simulink library "pmm"  (R2021b)
settings: Solver=VariableStepAuto  StartTime=0.0  StopTime=10.0  RelTol=1e-3
undefined symbols (not defined in the file or in its folder): ENUM_ACMAINRLYSTS_OPEN, ENUM_ACPRECHRGRLYSTS_OPEN, ENUM_B2VRLYSTA_OPEN, ENUM_BMSHVSTS_HVOPEN, ENUM_BRAKEPEDAL_RELEASED, ENUM_CACRLYDEM_CLOSE, ENUM_CACRLYSTS_OPEN, ENUM_CHRGFAULT_ACRLYFAIL, ENUM_CHRGFAULT_BCUHVFAIL, ENUM_CHRGFAULT_BCUNEGFAIL, ENUM_CHRGFAULT_BCUTIMEOUT, ENUM_CHRGFAULT_DCDCENABLE, ENUM_CHRGFAULT_DCDCRLYFAIL, ENUM_CHRGFAULT_HVILFAIL, ENUM_CHRGFAULT_PDUHVFAIL, ENUM_CHRGFAULT_RLYCHKFAIL, ENUM_DCDCEACPCURLYSTA_CLOSED, ENUM_DCDCEACPCURLYSTA_FAILTOCLOSE, ENUM_DCDCEACPCURLYSTA_OPEN, ENUM_DCDCEACPCURLYSTA_WELDED, ENUM_DCDCENABLESTS_READY, ENUM_DCDCRLYSTS_OPEN, ENUM_EHPSRLYDEM_CLOSE, ENUM_EHPSRLYSTS_OPEN, ENUM_FOGRLYENCMD_DISABLE, ENUM_GEARACTUALPOSN_D, ENUM_HVPWROFFREQ_POWEROFF, ENUM_KEYSTATUS_OFF, ENUM_KEYSTATUS_ON, ENUM_KEYSTATUS_START, ENUM_LOWBATTVOLTAGE_NORMAL, ENUM_LOWBATTVOLTAGE_POWERDOWN, ENUM_LOWBATTVOLTAGE_POWERUP, ENUM_MCUHVLOOP_POWEROFF, ENUM_MCUHVLOOPSTS_OPEN, ENUM_MCUMAINRLYSTS_OPEN, ENUM_MCUPRECHRGRLYSTS_OPEN, ENUM_PDFAULT_ACRLYOPEN, ENUM_PDFAULT_BCUDISABLE, ENUM_PDFAULT_DCDCDISABLE, ENUM_PDFAULT_DCDCRLYOPEN, ENUM_PDFAULT_EACDISABLE, ENUM_PDFAULT_EACRLYOPEN, ENUM_PDFAULT_EHPSDISABLE, ENUM_PDFAULT_EHPSRLYOPEN, ENUM_PDFAULT_MCUDISABLE, ENUM_PDFAULT_MCUDISCHRG, ENUM_PDFAULT_MCURLYOPEN, ENUM_PEUSELFCHKSTS_NOFAULT, ENUM_PLUGINSTS_NOPLUGIN, ENUM_PLUGINSTS_PLUGIN, ENUM_PMMMODE_DRIVE, ENUM_PMMMODE_LVBATCHRG, ENUM_PUSTATE_DCDCENABLE, ENUM_PUSTATE_EACPRESCHECK, ENUM_PUSTATE_EHPSENABLE, ENUM_PUSTATE_MCUENABLE, ENUM_PUSTATE_PDUMCURLYCLOSED, ENUM_PUSTATE_POWERUPFAIL, ENUM_TARGETGEAR_REVERSE ... (+126)
libraries: hcu_lib x45, simulink x5, ddm x1, dsc x1
(part 3 of 7)

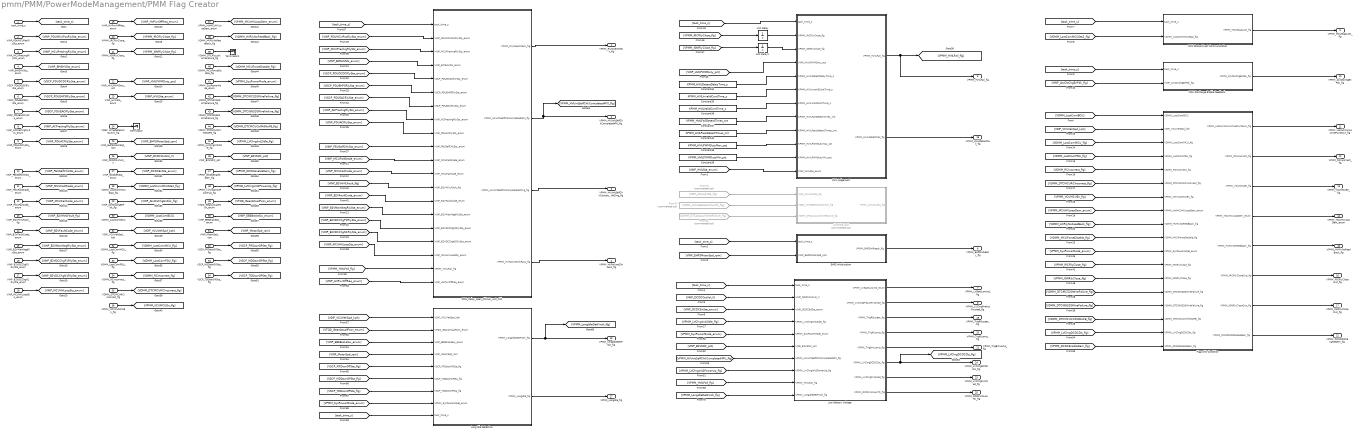
== system pmm/PMM/PowerModeManagement/PMM Flag Creator  ==
  task_time_s : Inport
  VINP_PDUMCUPosRlySta_enum : Inport  Port=2
  VINP_MCUPrechrgRlySts_enum : Inport  Port=3
  VINP_BMSHVSts_enum : Inport  Port=4
  VSCP_PDUDCDCRlySta_enum : Inport  Port=5
  VSCP_PDUEHPSRlySta_enum : Inport  Port=6
  VSCP_PDUEACRlySta_enum : Inport  Port=7
  VINP_ACPrechrgRlySts_enum : Inport  Port=8
  VINP_PDUACRlySta_enum : Inport  Port=9
  VINP_PEUSelfChkSts_enum : Inport  Port=10
  VINP_MCUFailGrade_enum : Inport  Port=11
  VINP_MCUFailCode_enum : Inport  Port=12
  VINP_B2VHVILFault_flg : Inport  Port=13
  VINP_B2VFaultCode_enum : Inport  Port=14
  VINP_B2VMainNegRlySta_enum : Inport  Port=15
  VINP_B2VDCChgP1RlySta_enum : Inport  Port=16
  VINP_B2VDCChgN1RlySta_enum : Inport  Port=17
  VINP_MCUHVLoopSts_enum : Inport  Port=18
  VINP_HVPwrOffReq_enum : Inport  Port=19
  VPMM_IRCRlyClose_flg : Inport  Port=20
  VPMM_IGNRlyClose_flg : Inport  Port=21
  VINP_HVILPWMDuty_pct : Inport  Port=22
  VINP_HVILSta_enum : Inport  Port=23
  VDSC_WineDetectorSwitch_flg : Inport  Port=24
  VINP_EHPSMotorSpd_rpm : Inport  Port=25
  VINP_DCDCOutVol_V : Inport  Port=26
  VINP_DCDCEnSta_enum : Inport  Port=27
  VDMM_LostComMCUSta2_flg : Inport  Port=28
  VINP_AtvDisChgEnFbk_flg : Inport  Port=29
  VDMM_LostComBCU : Inport  Port=30
  VDIP_VCUVehSpd_kph : Inport  Port=31
  VDMM_LostComMCU_flg : Inport  Port=32
  VDMM_LostComPDU_flg : Inport  Port=33
  VDMM_RCIncorrect_flg : Inport  Port=34
  VDMM_DTCMCURCIncorrect_flg : Inport  Port=35
  VPMM_InitVCUMCUEn_flg : Inport  Port=36
  VPMM_InitMCUHVLoopDem_enum : Inport  Port=37
  VDMM_HVRlyNoFeedBack_flg : Inport  Port=38
  VDMM_DTCAlcLockWireFailure_flg : Inport  Port=39
  VDMM_MCUForceDisable_flg : Inport  Port=40
  VPMM_SysPowerMode_enum : Inport  Port=41
  VDMM_DTCIRCS2GWireFailure_flg : Inport  Port=42
  VDMM_DTCIGNS2GWireFailure_flg : Inport  Port=43
  VDMM_DTCMCUCtrlMdNoFB_flg : Inport  Port=44
  VPMM_LVChrgIinit2Idle_flg : Inport  Port=45
  VINP_B2VSOC_pct : Inport  Port=46
  VPMM_DCDCEnableDem_flg : Inport  Port=47
  VPMM_LVChrgInit2PowerUp_flg : Inport  Port=48
  VTQD_GearActualPosn_enum : Inport  Port=49
  VINP_EBSBrakeSw_enum : Inport  Port=50
  VINP_MotorSpd_rpm : Inport  Port=51
  VSCP_FRDoorOPSta_flg : Inport  Port=52
  VSCP_MDDoorOPSta_flg : Inport  Port=53
  VSCP_TDDoorOPSta_flg : Inport  Port=54
  "Alcohole Lock " : Subsystem  Commented=on
  Constant34 : Constant  Value=KPMM_HVILDetectDelayTime_s
  Constant35 : Constant  Value=KPMM_HVILInvalidContTime_s
  Constant36 : Constant  Value=KPMM_HVILValidContTime_s
  Constant37 : Constant  Value=KPMM_HVILFailDetectTimes_cnt
  Constant38 : Constant  Value=KPMM_HVILPWMDutyMax_pct
  Constant39 : Constant  Value=KPMM_HVILPWMDutyMin_pct
  Constant40 : Constant  Value=KPMM_HVILPassDetectTimes_cnt
  EHPS Initialization : Subsystem
  Flag with Condition : Subsystem
  From24 : From  Commented=on  GotoTag=VDMM_DTCAlcLockWireFailure_flg
  From73 : From  Commented=on  GotoTag=VINP_AlcLockSta_flg
  From74 : From  Commented=on  GotoTag=VDSC_WineDetectorSwitch_flg
  HVIL Judgement : Subsystem
  Long Idle Detection : Subsystem
  Low Battery Voltage : Subsystem
  MCU Discharge Enable Feedback : Subsystem
  MCU Status2 Lost Communication : Subsystem
  PMM_Relay_open_Chk/HV_unit_Chk : Subsystem  Priority=1
      settings: AttributesFormatString=< Priority = %<Priority>>
  Terminator : Terminator
  Terminator1 : Terminator
  Unit Delay : UnitDelay  SampleTime=-1  HasFrameUpgradeWarning=on
  Unit Delay1 : UnitDelay  SampleTime=-1  HasFrameUpgradeWarning=on
  VPMM_RlyOpenCheck_flg : Outport
  VPMM_HVUnitSelfChkCompleted4PU_flg : Outport  Port=2
  VPMM_HVUnitSelfChkCompleted4Chrg_flg : Outport  Port=3
  VPMM_HVFailureChkPass_flg : Outport  Port=4
  VPMM_HVILFail_flg : Outport  Port=5  VectorParamsAs1DForOutWhenUnconnected=off
  VPMM_EHPSIniReady_flg : Outport  Port=6  VectorParamsAs1DForOutWhenUnconnected=off
  VPMM_LVBattLowInd_flg : Outport  Port=7
  VPMM_LVChrgPreActFinished_flg : Outport  Port=8
  VPMM_MCUSta2Lost_flg : Outport  Port=9  VectorParamsAs1DForOutWhenUnconnected=off
  VPMM_AtvDisChgEnFbk_flg : Outport  Port=10  VectorParamsAs1DForOutWhenUnconnected=off
  VPMM_LostHVComActivePwrDown_flg : Outport  Port=11
  VPMM_RCIncorrect_flg : Outport  Port=12  VectorParamsAs1DForOutWhenUnconnected=off
  VPMM_VCUMCUEn_flg : Outport  Port=13  VectorParamsAs1DForOutWhenUnconnected=off
  VPMM_MCUHVLoopDem_enum : Outport  Port=14  VectorParamsAs1DForOutWhenUnconnected=off
  VPMM_HVRlyNoFeedBack_flg : Outport  Port=15  VectorParamsAs1DForOutWhenUnconnected=off
  VPMM_IRCRlyCloseOut_flg : Outport  Port=16  VectorParamsAs1DForOutWhenUnconnected=off
  VPMM_IGNRlyCloseOut_flg : Outport  Port=17  VectorParamsAs1DForOutWhenUnconnected=off
  VPMM_HVILDetectFail_flg : Outport  Port=18  VectorParamsAs1DForOutWhenUnconnected=off
  VPMM_TrigRBuzeer_flg : Outport  Port=19
  VPMM_TrigRLamp_flg : Outport  Port=20
  VPMM_TrigBrkLamp_flg : Outport  Port=21
  VPMM_PMMDCDCEnableDem_flg : Outport  Port=22  VectorParamsAs1DForOutWhenUnconnected=off
  VPMM_LVChrgFinished_flg : Outport  Port=23
  VPMM_LVChrgDCDCDis_flg : Outport  Port=24
  VPMM_DCDCVolLowTO_flg : Outport  Port=25
  VPMM_LongIdleDetFinsh_flg : Outport  Port=26
  VPMM_LongIdle_flg : Outport  Port=27
  wires:
  HVIL Judgement/2(VPMM_HVILDetectFail_flg) -> VPMM_HVILDetectFail_flg/1
  [VINP_B2VHVILFault_flg] -> PMM_Relay_open_Chk/HV_unit_Chk/13(VINP_B2VHVILFault_flg)
  [task_time_s] -> PMM_Relay_open_Chk/HV_unit_Chk/1(task_time_s)
  [VINP_PEUSelfChkSts_enum] -> PMM_Relay_open_Chk/HV_unit_Chk/10(VINP_PEUSelfChkSts_enum)
  [VPMM_HVILFail_flg] -> PMM_Relay_open_Chk/HV_unit_Chk/19(VPMM_HVILFail_flg)
  [VINP_MCUHVLoopSts_enum] -> PMM_Relay_open_Chk/HV_unit_Chk/18(VINP_MCUHVLoopSts_enum)
  [VINP_B2VMainNegRlySta_enum] -> PMM_Relay_open_Chk/HV_unit_Chk/15(VINP_B2VMainNegRlySta_enum)
  [VINP_B2VFaultCode_enum] -> PMM_Relay_open_Chk/HV_unit_Chk/14(VINP_B2VFaultCode_enum)
  [VINP_B2VDCChgN1RlySta_enum] -> PMM_Relay_open_Chk/HV_unit_Chk/17(VINP_B2VDCChgN1RlySta_enum)
  [VINP_HVPwrOffReq_enum] -> PMM_Relay_open_Chk/HV_unit_Chk/20(VINP_HVPwrOffReq_enum)
  [VINP_B2VDCChgP1RlySta_enum] -> PMM_Relay_open_Chk/HV_unit_Chk/16(VINP_B2VDCChgP1RlySta_enum)
  [VINP_PDUACRlySta_enum] -> PMM_Relay_open_Chk/HV_unit_Chk/9(VINP_PDUACRlySta_enum)
  [VINP_MCUPrechrgRlySts_enum] -> PMM_Relay_open_Chk/HV_unit_Chk/3(VINP_MCUPrechrgRlySts_enum)
  PMM_Relay_open_Chk/HV_unit_Chk/3(VPMM_HVUnitSelfChkCompleted4Chrg_flg) -> VPMM_HVUnitSelfChkCompleted4Chrg_flg/1
  [VSCP_PDUEACRlySta_enum] -> PMM_Relay_open_Chk/HV_unit_Chk/7(VSCP_PDUEACRlySta_enum)
  [VINP_BMSHVSts_enum] -> PMM_Relay_open_Chk/HV_unit_Chk/4(VINP_BMSHVSts_enum)
  [VSCP_PDUDCDCRlySta_enum] -> PMM_Relay_open_Chk/HV_unit_Chk/5(VSCP_PDUDCDCRlySta_enum)
  [VINP_PDUMCUPosRlySta_enum] -> PMM_Relay_open_Chk/HV_unit_Chk/2(VINP_PDUMCUPosRlySta_enum)
  [VINP_ACPrechrgRlySts_enum] -> PMM_Relay_open_Chk/HV_unit_Chk/8(VINP_ACPrechrgRlySts_enum)
  [VSCP_PDUEHPSRlySta_enum] -> PMM_Relay_open_Chk/HV_unit_Chk/6(VSCP_PDUEHPSRlySta_enum)
  [VINP_MCUFailGrade_enum] -> PMM_Relay_open_Chk/HV_unit_Chk/11(VINP_MCUFailGrade_enum)
  PMM_Relay_open_Chk/HV_unit_Chk/1(VPMM_RlyOpenCheck_flg) -> VPMM_RlyOpenCheck_flg/1
  PMM_Relay_open_Chk/HV_unit_Chk/2(VPMM_HVUnitSelfChkCompleted4PU_flg) -> [VPMM_HVUnitSelfChkCompleted4PU_flg], VPMM_HVUnitSelfChkCompleted4PU_flg/1
  [VINP_MCUFailCode_enum] -> PMM_Relay_open_Chk/HV_unit_Chk/12(VINP_MCUFailCode_enum)
  PMM_Relay_open_Chk/HV_unit_Chk/4(VPMM_HVFailureChkPass_flg) -> VPMM_HVFailureChkPass_flg/1
  task_time_s/1 -> [task_time_s]
  VINP_PDUMCUPosRlySta_enum/1 -> [VINP_PDUMCUPosRlySta_enum]
  VINP_MCUPrechrgRlySts_enum/1 -> [VINP_MCUPrechrgRlySts_enum]
  VINP_BMSHVSts_enum/1 -> [VINP_BMSHVSts_enum]
  VSCP_PDUDCDCRlySta_enum/1 -> [VSCP_PDUDCDCRlySta_enum]
  VSCP_PDUEHPSRlySta_enum/1 -> [VSCP_PDUEHPSRlySta_enum]
  VSCP_PDUEACRlySta_enum/1 -> [VSCP_PDUEACRlySta_enum]
  VINP_ACPrechrgRlySts_enum/1 -> [VINP_ACPrechrgRlySts_enum]
  VINP_PDUACRlySta_enum/1 -> [VINP_PDUACRlySta_enum]
  VINP_PEUSelfChkSts_enum/1 -> [VINP_PEUSelfChkSts_enum]
  VINP_MCUFailGrade_enum/1 -> [VINP_MCUFailGrade_enum]
  VINP_MCUFailCode_enum/1 -> [VINP_MCUFailCode_enum]
  VINP_B2VHVILFault_flg/1 -> [VINP_B2VHVILFault_flg]
  VINP_B2VFaultCode_enum/1 -> [VINP_B2VFaultCode_enum]
  VINP_B2VMainNegRlySta_enum/1 -> [VINP_B2VMainNegRlySta_enum]
  VINP_B2VDCChgP1RlySta_enum/1 -> [VINP_B2VDCChgP1RlySta_enum]
  VINP_B2VDCChgN1RlySta_enum/1 -> [VINP_B2VDCChgN1RlySta_enum]
  VINP_MCUHVLoopSts_enum/1 -> [VINP_MCUHVLoopSts_enum]
  VINP_HVPwrOffReq_enum/1 -> [VINP_HVPwrOffReq_enum]
  [task_time_s] -> HVIL Judgement/1(task_time_s)
  [VPMM_IRCRlyClose_flg] -> Unit Delay/1
  Unit Delay1/1 -> HVIL Judgement/3(VPMM_IGNRlyClose_flg)
  [VPMM_IGNRlyClose_flg] -> Unit Delay1/1
  [VINP_HVILPWMDuty_pct] -> HVIL Judgement/4(VINP_HVILPWMDuty_pct)
  Constant36/1 -> HVIL Judgement/7(KPMM_HVILValidContTime_s)
  Constant40/1 -> HVIL Judgement/9(KPMM_HVILPassDetectTimes_cnt)
  Constant37/1 -> HVIL Judgement/8(KPMM_HVILFailDetectTimes_cnt)
  Unit Delay/1 -> HVIL Judgement/2(VPMM_IRCRlyClose_flg)
  Constant35/1 -> HVIL Judgement/6(KPMM_HVILInvalidContTime_s)
  Constant38/1 -> HVIL Judgement/10(KPMM_HVILPWMDutyMax_pct)
  Constant34/1 -> HVIL Judgement/5(KPMM_HVILDetectDelayTime_s)
  Constant39/1 -> HVIL Judgement/11(KPMM_HVILPWMDutyMin_pct)
  HVIL Judgement/1(VPMM_HVILFail_flg) -> [VPMM_HVILFail_flg], VPMM_HVILFail_flg/1
  [VINP_HVILSta_enum] -> HVIL Judgement/12(VINP_HVILSta_enum)
  VPMM_IRCRlyClose_flg/1 -> [VPMM_IRCRlyClose_flg]
  VPMM_IGNRlyClose_flg/1 -> [VPMM_IGNRlyClose_flg]
  VINP_HVILPWMDuty_pct/1 -> [VINP_HVILPWMDuty_pct]
  VINP_HVILSta_enum/1 -> [VINP_HVILSta_enum]
  From73/1 -> "Alcohole Lock "/1(VINP_AlcLockSta_flg)
  From74/1 -> "Alcohole Lock "/2(VDSC_WineDetectorSwitch_flg)
  VDSC_WineDetectorSwitch_flg/1 -> Terminator/1
  EHPS Initialization/1(VPMM_EHPSIniReady_flg) -> VPMM_EHPSIniReady_flg/1
  [task_time_s] -> EHPS Initialization/1(task_time_s)
  [VINP_EHPSMotorSpd_rpm] -> EHPS Initialization/2(VINP_EHPSMotorSpd_rpm)
  VINP_EHPSMotorSpd_rpm/1 -> [VINP_EHPSMotorSpd_rpm]
  Low Battery Voltage/1(VPMM_LVBattLowInd_enum) -> VPMM_LVBattLowInd_flg/1
  [task_time_s] -> Low Battery Voltage/1(task_time_s)
  VINP_DCDCEnSta_enum/1 -> [VINP_DCDCEnSta_enum]
  VINP_DCDCOutVol_V/1 -> [VINP_DCDCOutVol_V]
  [VINP_DCDCOutVol_V] -> Low Battery Voltage/2(VINP_DCDCOutVol_V)
  [VINP_DCDCEnSta_enum] -> Low Battery Voltage/3(VINP_DCDCEnSta_enum)
  MCU Status2 Lost Communication/1(VPMM_MCUSta2Lost_flg) -> VPMM_MCUSta2Lost_flg/1
  VDMM_LostComMCUSta2_flg/1 -> [VDMM_LostComMCUSta2_flg]
  [task_time_s] -> MCU Status2 Lost Communication/1(task_time_s)
  [VDMM_LostComMCUSta2_flg] -> MCU Status2 Lost Communication/2(VDMM_LostComMCUSta2_flg)
  MCU Discharge Enable Feedback/1(VPMM_AtvDisChgEnFbk_flg) -> VPMM_AtvDisChgEnFbk_flg/1
  [task_time_s] -> MCU Discharge Enable Feedback/1(task_time_s)
  [VINP_AtvDisChgEnFbk_flg] -> MCU Discharge Enable Feedback/2(VINP_AtvDisChgEnFbk_flg)
  VINP_AtvDisChgEnFbk_flg/1 -> [VINP_AtvDisChgEnFbk_flg]
  Flag with Condition/1(VPMM_LostHVComActivePwrDown_flg) -> VPMM_LostHVComActivePwrDown_flg/1
  Flag with Condition/2(VPMM_RCIncorrect_flg) -> VPMM_RCIncorrect_flg/1
  Flag with Condition/3(VPMM_VCUMCUEn_flg) -> VPMM_VCUMCUEn_flg/1
  Flag with Condition/4(VPMM_MCUHVLoopDem_enum) -> VPMM_MCUHVLoopDem_enum/1
  VDMM_LostComBCU/1 -> [VDMM_LostComBCU]
  VDMM_DTCMCURCIncorrect_flg/1 -> [VDMM_DTCMCURCIncorrect_flg]
  VDMM_LostComPDU_flg/1 -> [VDMM_LostComPDU_flg]
  VPMM_InitVCUMCUEn_flg/1 -> [VPMM_VCUMCUEn_flg]
  VPMM_InitMCUHVLoopDem_enum/1 -> [VPMM_MCUHVLoopDem_enum]
  VDMM_LostComMCU_flg/1 -> [VDMM_LostComMCU_flg]
  VDMM_RCIncorrect_flg/1 -> [VDMM_RCIncorrect_flg]
  VDIP_VCUVehSpd_kph/1 -> [VDIP_VCUVehSpd_kph]
  [VDMM_LostComBCU] -> Flag with Condition/1(VDMM_LostComBCU)
  [VDIP_VCUVehSpd_kph] -> Flag with Condition/2(VDIP_VCUVehSpd_kph)
  [VDMM_LostComMCU_flg] -> Flag with Condition/3(VDMM_LostComMCU_flg)
  [VDMM_LostComPDU_flg] -> Flag with Condition/4(VDMM_LostComPDU_flg)
  [VDMM_RCIncorrect_flg] -> Flag with Condition/5(VDMM_RCIncorrect_flg)
  [VDMM_DTCMCURCIncorrect_flg] -> Flag with Condition/6(VDMM_DTCMCURCIncorrect_flg)
  [VPMM_VCUMCUEn_flg] -> Flag with Condition/7(VPMM_InitVCUMCUEn_flg)
  [VPMM_MCUHVLoopDem_enum] -> Flag with Condition/8(VPMM_InitMCUHVLoopDem_enum)
  [VDMM_HVRlyNoFeedBack_flg] -> Flag with Condition/9(VDMM_HVRlyNoFeedBack_flg)
  Flag with Condition/5(VPMM_HVRlyNoFeedBack_flg) -> VPMM_HVRlyNoFeedBack_flg/1
  VDMM_HVRlyNoFeedBack_flg/1 -> [VDMM_HVRlyNoFeedBack_flg]
  From24/1 -> "Alcohole Lock "/3(VDMM_DTCAlcLockWireFailure_flg)
  VDMM_DTCAlcLockWireFailure_flg/1 -> Terminator1/1
  VDMM_MCUForceDisable_flg/1 -> [VDMM_MCUForceDisable_flg]
  [VDMM_MCUForceDisable_flg] -> Flag with Condition/10(VDMM_MCUForceDisable_flg)
  VPMM_SysPowerMode_enum/1 -> [VPMM_SysPowerMode_enum]
  [VPMM_SysPowerMode_enum] -> Flag with Condition/11(VPMM_SysPowerMode_enum)
  VDMM_DTCIRCS2GWireFailure_flg/1 -> [VDMM_DTCIRCS2GWireFailure_flg]
  VDMM_DTCIGNS2GWireFailure_flg/1 -> [VDMM_DTCIGNS2GWireFailure_flg]
  Flag with Condition/6(VPMM_IRCRlyCloseOut_flg) -> VPMM_IRCRlyCloseOut_flg/1
  Flag with Condition/7(VPMM_IGNRlyCloseOut_flg) -> VPMM_IGNRlyCloseOut_flg/1
  [VPMM_IRCRlyClose_flg] -> Flag with Condition/12(VPMM_IRCRlyClose_flg)
  [VPMM_IGNRlyClose_flg] -> Flag with Condition/13(VPMM_IGNRlyClose_flg)
  [VDMM_DTCIRCS2GWireFailure_flg] -> Flag with Condition/14(VDMM_DTCIRCS2GWireFailure_flg)
  [VDMM_DTCIGNS2GWireFailure_flg] -> Flag with Condition/15(VDMM_DTCIGNS2GWireFailure_flg)
  VDMM_DTCMCUCtrlMdNoFB_flg/1 -> [VDMM_DTCMCUCtrlMdNoFB_flg]
  [VDMM_DTCMCUCtrlMdNoFB_flg] -> Flag with Condition/16(VDMM_DTCMCUCtrlMdNoFB_flg)
  Low Battery Voltage/2(VPMM_LVChrgPreActFinished_flg) -> VPMM_LVChrgPreActFinished_flg/1
  [VPMM_LVChrgIinit2Idle_flg] -> Low Battery Voltage/4(VPMM_LVChrgIinit2Idle_flg)
  VPMM_LVChrgIinit2Idle_flg/1 -> [VPMM_LVChrgIinit2Idle_flg]
  [VPMM_SysPowerMode_enum] -> Low Battery Voltage/5(VPMM_SysPowerMode_enum)
  Low Battery Voltage/5(VPMM_TrigBrkLamp_flg) -> VPMM_TrigBrkLamp_flg/1
  Low Battery Voltage/4(VPMM_TrigRLamp_flg) -> VPMM_TrigRLamp_flg/1
  Low Battery Voltage/3(VPMM_TrigRBuzeer_flg) -> VPMM_TrigRBuzeer_flg/1
  [VINP_B2VSOC_pct] -> Low Battery Voltage/6(VINP_B2VSOC_pct)
  VINP_B2VSOC_pct/1 -> [VINP_B2VSOC_pct]
  [VPMM_HVUnitSelfChkCompleted4PU_flg] -> Low Battery Voltage/7(VPMM_HVUnitSelfChkCompleted4PU_flg)
  Low Battery Voltage/6(VPMM_LVChrgDCDCDis_flg) -> [VPMM_LVChrgDCDCDis_flg], VPMM_LVChrgDCDCDis_flg/1
  [VPMM_LVChrgDCDCDis_flg] -> Flag with Condition/17(VPMM_LVChrgDCDCDis_flg)
  VPMM_DCDCEnableDem_flg/1 -> [VPMM_DCDCEnableDem_flg]
  [VPMM_DCDCEnableDem_flg] -> Flag with Condition/18(VPMM_DCDCEnableDem_flg)
  Flag with Condition/8(VPMM_PMMDCDCEnableDem_flg) -> VPMM_PMMDCDCEnableDem_flg/1
  Low Battery Voltage/7(VPMM_LVChrgFinished_flg) -> VPMM_LVChrgFinished_flg/1
  Low Battery Voltage/8(VPMM_DCDCVolLowTO_flg) -> VPMM_DCDCVolLowTO_flg/1
  VPMM_LVChrgInit2PowerUp_flg/1 -> [VPMM_LVChrgInit2PowerUp_flg]
  [VPMM_LVChrgInit2PowerUp_flg] -> Low Battery Voltage/8(VPMM_LVChrgInit2PowerUp_flg)
  [VPMM_HVILFail_flg] -> Low Battery Voltage/9(VPMM_HVILFail_flg)
  [VDIP_VCUVehSpd_kph] -> Long Idle Detection/1(VDIP_VCUVehSpd_kph)
  [VTQD_GearActualPosn_enum] -> Long Idle Detection/2(VTQD_GearActualPosn_enum)
  [VINP_EBSBrakeSw_enum] -> Long Idle Detection/3(VINP_EBSBrakeSw_enum)
  [VINP_MotorSpd_rpm] -> Long Idle Detection/4(VINP_MotorSpd_rpm)
  [VSCP_FRDoorOPSta_flg] -> Long Idle Detection/5(VSCP_FRDoorOPSta_flg)
  [VSCP_MDDoorOPSta_flg] -> Long Idle Detection/6(VSCP_MDDoorOPSta_flg)
  [VSCP_TDDoorOPSta_flg] -> Long Idle Detection/7(VSCP_TDDoorOPSta_flg)
  [task_time_s] -> Long Idle Detection/9(task_time_s)
  Long Idle Detection/1(VPMM_LongIdleDetFinsh_flg) -> [VPMM_LongIdleDetFinsh_flg], VPMM_LongIdleDetFinsh_flg/1
  VTQD_GearActualPosn_enum/1 -> [VTQD_GearActualPosn_enum]
  VINP_EBSBrakeSw_enum/1 -> [VINP_EBSBrakeSw_enum]
  VINP_MotorSpd_rpm/1 -> [VINP_MotorSpd_rpm]
  VSCP_FRDoorOPSta_flg/1 -> [VSCP_FRDoorOPSta_flg]
  VSCP_MDDoorOPSta_flg/1 -> [VSCP_MDDoorOPSta_flg]
  VSCP_TDDoorOPSta_flg/1 -> [VSCP_TDDoorOPSta_flg]
  [VPMM_LongIdleDetFinsh_flg] -> Low Battery Voltage/10(VPMM_LongIdleDetFinsh_flg)
  Long Idle Detection/2(VPMM_LongIdle_flg) -> VPMM_LongIdle_flg/1
  [VPMM_SysPowerMode_enum] -> Long Idle Detection/8(VPMM_SysPowerMode_enum)

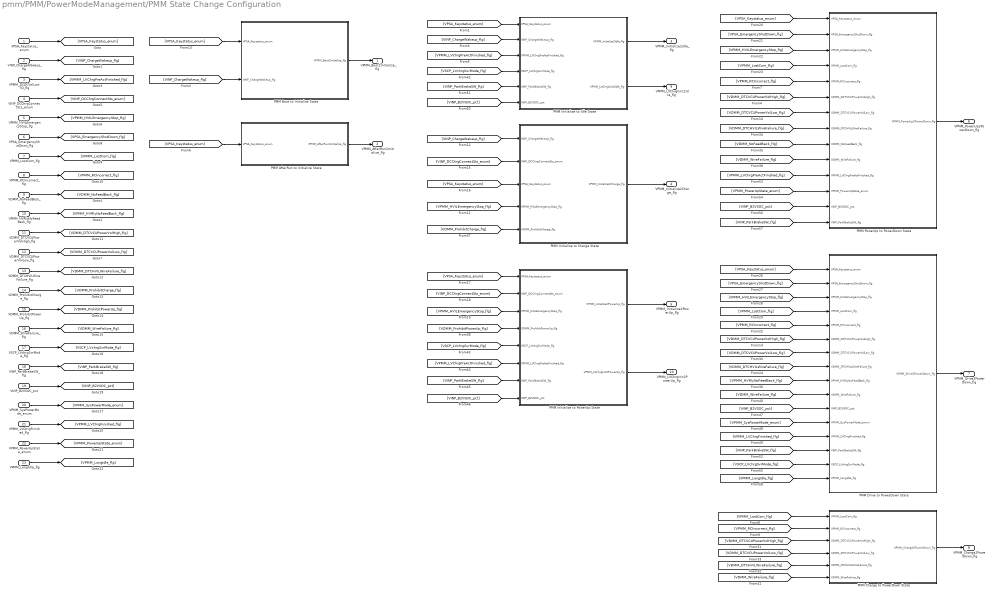
== system pmm/PMM/PowerModeManagement/PMM State Change Configuration ==
  VPSA_Keystatus_enum : Inport
  VINP_ChargeWakeup_flg : Inport  Port=2
  VPMM_DCDCVolLowTO_flg : Inport  Port=3
  VINP_DCChrgConnectSts_enum : Inport  Port=4
  VPMM_HVILEmergencyStop_flg : Inport  Port=5
  VPSA_EmergencyShutDown_flg : Inport  Port=6
  VPMM_LostCom_flg : Inport  Port=7
  VPMM_RCIncorrect_flg : Inport  Port=8
  VDMM_NoFeedBack_flg : Inport  Port=9
  VPMM_HVRlyNoFeedBack_flg : Inport  Port=10
  VDMM_DTCVCUPowerVolHigh_flg : Inport  Port=11
  VDMM_DTCVCUPowerVolLow_flg : Inport  Port=12
  VDMM_DTCHVILWireFailure_flg : Inport  Port=13
  VDMM_ProhibitCharge_flg : Inport  Port=14
  VDMM_ProhibitPowerUp_flg : Inport  Port=15
  VDMM_WireFailure_flg : Inport  Port=16
  VSCP_LVchrgSvrMode_flg : Inport  Port=17
  VINP_ParkBrakeSW_flg : Inport  Port=18
  VINP_B2VSOC_pct : Inport  Port=19
  VPMM_SysPowerMode_enum : Inport  Port=20
  VPMM_LVChrgFinished_flg : Inport  Port=21
  VPMM_PowerUpState_enum : Inport  Port=22
  VPMM_LongIdle_flg : Inport  Port=23
  PMM AfterRun to Initialize State : Subsystem
  PMM Boot to Initialize State : Subsystem
  PMM Charge to PowerDown State : Subsystem
  PMM Drive to PowerDown State : Subsystem
  PMM Initialize to Charge State : Subsystem
  PMM Initialize to Idle State : Subsystem
  PMM Initialize to PowerUp State : Subsystem
  PMM PowerUp to PowerDown State : Subsystem
  VPMM_Boot2Initialize_flg : Outport
  VPMM_AfterRun2Initialize_flg : Outport  Port=2
  VPMM_Initialize2Idle_flg : Outport  Port=3
  VPMM_Initialize2Charge_flg : Outport  Port=4
  VPMM_Initialize2PowerUp_flg : Outport  Port=5
  VPMM_PowerUp2PowerDown_flg : Outport  Port=6
  VPMM_Drive2PowerDown_flg : Outport  Port=7
  VPMM_Charge2PowerDown_flg : Outport  Port=8
  VPMM_LVChrgIinit2Idle_flg : Outport  Port=9
  VPMM_LVChrgInit2PowerUp_flg : Outport  Port=10
  wires:
  [VPSA_EmergencyShutDown_flg] -> PMM PowerUp to PowerDown State/2(VPSA_EmergencyShutDown_flg)
  PMM AfterRun to Initialize State/1(VPMM_AfterRun2Initialize_flg) -> VPMM_AfterRun2Initialize_flg/1
  [VPMM_HVILEmergencyStop_flg] -> PMM Initialize to Charge State/4(VPMM_HVILEmergencyStop_flg)
  PMM Initialize to PowerUp State/1(VPMM_Initialize2PowerUp_flg) -> VPMM_Initialize2PowerUp_flg/1
  [VPSA_EmergencyShutDown_flg] -> PMM Drive to PowerDown State/2(VPSA_EmergencyShutDown_flg)
  [VINP_DCChrgConnectSts_enum] -> PMM Initialize to Charge State/2(VINP_DCChrgConnectSts_enum)
  [VPMM_HVILEmergencyStop_flg] -> PMM PowerUp to PowerDown State/3(VPMM_HVILEmergencyStop_flg)
  [VPMM_LostCom_flg] -> PMM Drive to PowerDown State/4(VPMM_LostCom_flg)
  [VPMM_LostCom_flg] -> PMM Charge to PowerDown State/1(VPMM_LostCom_flg)
  [VINP_ChargeWakeup_flg] -> PMM Initialize to Idle State/2(VINP_ChargeWakeup_flg)
  [VPSA_Keystatus_enum] -> PMM Drive to PowerDown State/1(VPSA_Keystatus_enum)
  PMM Charge to PowerDown State/1(VPMM_Charge2PowerDown_flg) -> VPMM_Charge2PowerDown_flg/1
  [VPMM_HVILEmergencyStop_flg] -> PMM Drive to PowerDown State/3(VPMM_HVILEmergencyStop_flg)
  PMM Boot to Initialize State/1(VPMM_Boot2Initialize_flg) -> VPMM_Boot2Initialize_flg/1
  [VPMM_RCIncorrect_flg] -> PMM Charge to PowerDown State/2(VPMM_RCIncorrect_flg)
  [VPMM_RCIncorrect_flg] -> PMM Drive to PowerDown State/5(VPMM_RCIncorrect_flg)
  [VINP_ChargeWakeup_flg] -> PMM Boot to Initialize State/2(VINP_ChargeWakeup_flg)
  [VPMM_LVChrgPreActFinished_flg] -> PMM Initialize to Idle State/3(VPMM_LVChrgPreActFinished_flg)
  PMM Initialize to Idle State/1(VPMM_Initialize2Idle_flg) -> VPMM_Initialize2Idle_flg/1
  [VPMM_LostCom_flg] -> PMM PowerUp to PowerDown State/4(VPMM_LostCom_flg)
  [VINP_ChargeWakeup_flg] -> PMM Initialize to Charge State/1(VINP_ChargeWakeup_flg)
  [VPSA_Keystatus_enum] -> PMM Initialize to Charge State/3(VPSA_Keystatus_enum)
  PMM Initialize to Charge State/1(VPMM_Initialize2Charge_flg) -> VPMM_Initialize2Charge_flg/1
  [VPMM_HVILEmergencyStop_flg] -> PMM Initialize to PowerUp State/3(VPMM_HVILEmergencyStop_flg)
  [VPSA_Keystatus_enum] -> PMM Boot to Initialize State/1(VPSA_Keystatus_enum)
  PMM Drive to PowerDown State/1(VPMM_Drive2PowerDown_flg) -> VPMM_Drive2PowerDown_flg/1
  [VPSA_Keystatus_enum] -> PMM Initialize to Idle State/1(VPSA_Keystatus_enum)
  [VINP_DCChrgConnectSts_enum] -> PMM Initialize to PowerUp State/2(VINP_DCChrgConnectSts_enum)
  [VPSA_Keystatus_enum] -> PMM Initialize to PowerUp State/1(VPSA_Keystatus_enum)
  [VPSA_Keystatus_enum] -> PMM AfterRun to Initialize State/1(VPSA_Keystatus_enum)
  PMM PowerUp to PowerDown State/1(VPMM_PowerUp2PowerDown_flg) -> VPMM_PowerUp2PowerDown_flg/1
  [VPSA_Keystatus_enum] -> PMM PowerUp to PowerDown State/1(VPSA_Keystatus_enum)
  VPSA_Keystatus_enum/1 -> [VPSA_Keystatus_enum]
  VINP_ChargeWakeup_flg/1 -> [VINP_ChargeWakeup_flg]
  VPMM_DCDCVolLowTO_flg/1 -> [VPMM_LVChrgPreActFinished_flg]
  VINP_DCChrgConnectSts_enum/1 -> [VINP_DCChrgConnectSts_enum]
  VPMM_HVILEmergencyStop_flg/1 -> [VPMM_HVILEmergencyStop_flg]
  VPSA_EmergencyShutDown_flg/1 -> [VPSA_EmergencyShutDown_flg]
  VPMM_LostCom_flg/1 -> [VPMM_LostCom_flg]
  VPMM_RCIncorrect_flg/1 -> [VPMM_RCIncorrect_flg]
  [VPMM_RCIncorrect_flg] -> PMM PowerUp to PowerDown State/5(VPMM_RCIncorrect_flg)
  VPMM_HVRlyNoFeedBack_flg/1 -> [VPMM_HVRlyNoFeedBack_flg]
  VDMM_NoFeedBack_flg/1 -> [VDMM_NoFeedBack_flg]
  VDMM_DTCVCUPowerVolHigh_flg/1 -> [VDMM_DTCVCUPowerVolHigh_flg]
  VDMM_DTCVCUPowerVolLow_flg/1 -> [VDMM_DTCVCUPowerVolLow_flg]
  [VDMM_DTCVCUPowerVolLow_flg] -> PMM PowerUp to PowerDown State/7(VDMM_DTCVCUPowerVolLow_flg)
  [VDMM_DTCVCUPowerVolHigh_flg] -> PMM PowerUp to PowerDown State/6(VDMM_DCTVCUPowerVolHigh_flg)
  VDMM_DTCHVILWireFailure_flg/1 -> [VDMM_DTCHVILWireFailure_flg]
  [VDMM_DTCVCUPowerVolHigh_flg] -> PMM Drive to PowerDown State/6(VDMM_DTCVCUPowerVolHigh_flg)
  [VDMM_DTCVCUPowerVolLow_flg] -> PMM Drive to PowerDown State/7(VDMM_DTCVCUPowerVolLow_flg)
  [VDMM_DTCHVILWireFailure_flg] -> PMM Drive to PowerDown State/8(VDMM_DTCHVILWireFailure_flg)
  [VDMM_DTCVCUPowerVolHigh_flg] -> PMM Charge to PowerDown State/3(VDMM_DTCVCUPowerVolHigh_flg)
  [VDMM_DTCVCUPowerVolLow_flg] -> PMM Charge to PowerDown State/4(VDMM_DTCVCUPowerVolLow_flg)
  [VDMM_DTCHVILWireFailure_flg] -> PMM Charge to PowerDown State/5(VDMM_DTCHVILWireFailure_flg)
  [VDMM_DTCHVILWireFailure_flg] -> PMM PowerUp to PowerDown State/8(VDMM_DTCHVILWireFailure_flg)
  [VDMM_NoFeedBack_flg] -> PMM PowerUp to PowerDown State/9(VDMM_NoFeedBack_flg)
  [VPMM_HVRlyNoFeedBack_flg] -> PMM Drive to PowerDown State/9(VPMM_HVRlyNoFeedBack_flg)
  VDMM_ProhibitCharge_flg/1 -> [VDMM_ProhibitCharge_flg]
  [VDMM_ProhibitCharge_flg] -> PMM Initialize to Charge State/5(VDMM_ProhibitCharge_flg)
  VDMM_ProhibitPowerUp_flg/1 -> [VDMM_ProhibitPowerUp_flg]
  [VDMM_ProhibitPowerUp_flg] -> PMM Initialize to PowerUp State/4(VDMM_ProhibitPowerUp_flg)
  VDMM_WireFailure_flg/1 -> [VDMM_WireFailure_flg]
  [VDMM_WireFailure_flg] -> PMM PowerUp to PowerDown State/10(VDMM_WireFailure_flg)
  [VDMM_WireFailure_flg] -> PMM Drive to PowerDown State/10(VDMM_WireFailure_flg)
  [VDMM_WireFailure_flg] -> PMM Charge to PowerDown State/6(VDMM_WireFailure_flg)
  VSCP_LVchrgSvrMode_flg/1 -> [VSCP_LVchrgSvrMode_flg]
  [VSCP_LVchrgSvrMode_flg] -> PMM Initialize to Idle State/4(VSCP_LVchrgSvrMode_flg)
  PMM Initialize to Idle State/2(VPMM_LVChrgIinit2Idle_flg) -> VPMM_LVChrgIinit2Idle_flg/1
  [VSCP_LVchrgSvrMode_flg] -> PMM Initialize to PowerUp State/5(VSCP_LVchrgSvrMode_flg)
  [VPMM_LVChrgPreActFinished_flg] -> PMM Initialize to PowerUp State/6(VPMM_LVChrgPreActFinished_flg)
  [VINP_B2VSOC_pct] -> PMM Initialize to PowerUp State/8(VINP_B2VSOC_pct)
  [VINP_ParkBrakeSW_flg] -> PMM Initialize to PowerUp State/7(VINP_ParkBrakeSW_flg)
  VINP_ParkBrakeSW_flg/1 -> [VINP_ParkBrakeSW_flg]
  VINP_B2VSOC_pct/1 -> [VINP_B2VSOC_pct]
  PMM Initialize to PowerUp State/2(VPMM_LVChrgInit2PowerUp_flg) -> VPMM_LVChrgInit2PowerUp_flg/1
  [VINP_B2VSOC_pct] -> PMM Drive to PowerDown State/11(VINP_B2VSOC_pct)
  VPMM_SysPowerMode_enum/1 -> [VPMM_SysPowerMode_enum]
  [VPMM_SysPowerMode_enum] -> PMM Drive to PowerDown State/12(VPMM_SysPowerMode_enum)
  VPMM_LVChrgFinished_flg/1 -> [VPMM_LVChrgFinished_flg]
  [VPMM_LVChrgFinished_flg] -> PMM Drive to PowerDown State/13(VPMM_LVChrgFinished_flg)
  [VINP_ParkBrakeSW_flg] -> PMM Initialize to Idle State/5(VINP_ParkBrakeSW_flg)
  [VINP_B2VSOC_pct] -> PMM Initialize to Idle State/6(VINP_B2VSOC_pct)
  [VINP_ParkBrakeSW_flg] -> PMM Drive to PowerDown State/14(VINP_ParkBrakeSW_flg)
  [VPMM_LVChrgPreActFinished_flg] -> PMM PowerUp to PowerDown State/11(VPMM_LVChrgPreActFinished_flg)
  VPMM_PowerUpState_enum/1 -> [VPMM_PowerUpState_enum]
  [VPMM_PowerUpState_enum] -> PMM PowerUp to PowerDown State/12(VPMM_PowerUpState_enum)
  [VSCP_LVchrgSvrMode_flg] -> PMM Drive to PowerDown State/15(VSCP_LVchrgSvrMode_flg)
  [VINP_B2VSOC_pct] -> PMM PowerUp to PowerDown State/13(VINP_B2VSOC_pct)
  [VINP_ParkBrakeSW_flg] -> PMM PowerUp to PowerDown State/14(VINP_ParkBrakeSW_flg)
  VPMM_LongIdle_flg/1 -> [VPMM_LongIdle_flg]
  [VPMM_LongIdle_flg] -> PMM Drive to PowerDown State/16(VPMM_LongIdle_flg)

== system pmm/PMM/PowerModeManagement/PMM Switch Enum Creator ==
  VPMM_InitPowerUpState_enum : Inport
  task_time_s : Inport  Port=2
  VPMM_MCUPrechrgProc_flg : Inport  Port=3
  VPMM_MCUEnableProc_flg : Inport  Port=4
  VPMM_DCDCEnableProc_flg : Inport  Port=5
  VPMM_EHPSEnableProc_flg : Inport  Port=6
  VPMM_CACPresReadyProc_flg : Inport  Port=7
  VPMM_InitPowerDownFault_enum : Inport  Port=8
  VPMM_InitChrgFault_enum : Inport  Port=9
  ChrgFault_SW : Subsystem
  Constant44 : Constant  Value=KPMM_TwoSysSwOFF_flg
  Constant49 : Constant  Value=ENUM_PUSTATE_PDUMCURLYCLOSED
  Constant50 : Constant  Value=ENUM_PUSTATE_MCUENABLE
  Constant51 : Constant  Value=ENUM_PUSTATE_DCDCENABLE
  Constant52 : Constant  Value=ENUM_PUSTATE_EHPSENABLE
  Constant53 : Constant  Value=ENUM_PUSTATE_EACPRESCHECK
  Constant54 : Constant  Value=KPMM_StaSwTime_s
  Data Type Conversion : DataTypeConversion  OutDataTypeStr=uint32
  Data Type Conversion28 : DataTypeConversion
  Data Type Conversion29 : DataTypeConversion
  Data Type Conversion30 : DataTypeConversion
  Divide : Product  Inputs=*/
  Floor : Rounding
  PowerDownFault_SW : Subsystem
  PowerUpState_SW : Subsystem
  Switch2 : Switch  Criteria=u2 > Threshold
  cycle time setting : Stateflow chart  TreatAsAtomicUnit=on
  VPMM_PowerUpState_enum : Outport  VectorParamsAs1DForOutWhenUnconnected=off
  VPMM_PowerDownFault_enum : Outport  Port=2  VectorParamsAs1DForOutWhenUnconnected=off
  VPMM_ChrgFault_enum : Outport  Port=3  VectorParamsAs1DForOutWhenUnconnected=off
  wires:
  Constant52/1 -> PowerUpState_SW/10(d_enum)
  PowerDownFault_SW/1(OUT_) -> Data Type Conversion29/1
  [VPMM_PowerDownFault_enum] -> PowerDownFault_SW/1(VPMM_PowerDownFault_enum)
  cycle time setting/1(trig()) -> PowerUpState_SW/Trigger
  Data Type Conversion29/1 -> VPMM_PowerDownFault_enum/1  "VPMM_PowerDownFault_enum"
  Constant51/1 -> PowerUpState_SW/9(c_enum)
  Divide/1 -> Floor/1
  [VPMM_DCDCEnableProc_flg] -> PowerUpState_SW/4(c_in)
  [VPMM_ChrgFault_enum] -> ChrgFault_SW/1(VPMM_ChrgFault_enum)
  [VPMM_MCUPrechrgProc_flg] -> PowerUpState_SW/2(a_in)
  [VPMM_CACPresReadyProc_flg] -> PowerUpState_SW/6(e_in)
  Constant50/1 -> PowerUpState_SW/8(b_enum)
  [VPMM_MCUEnableProc_flg] -> PowerUpState_SW/3(b_in)
  Constant53/1 -> PowerUpState_SW/11(e_enum)
  Data Type Conversion30/1 -> VPMM_ChrgFault_enum/1  "VPMM_ChrgFault_enum"
  [task_time_s] -> PowerDownFault_SW/2(task_time_s)
  [VPMM_EHPSEnableProc_flg] -> PowerUpState_SW/5(d_in)
  Constant44/1 -> Switch2/2
  [task_time_s] -> Divide/2
  Floor/1 -> Data Type Conversion/1
  [VPMM_PowerUpState_enum] -> PowerUpState_SW/1(Sys_in)
  Constant54/1 -> Divide/1
  [task_time_s] -> ChrgFault_SW/2(task_time_s)
  Data Type Conversion28/1 -> VPMM_PowerUpState_enum/1  "VPMM_PowerUpState_enum"
  ChrgFault_SW/1(OUT_) -> Data Type Conversion30/1
  PowerUpState_SW/1(OUT_enum) -> Switch2/3
  Constant49/1 -> PowerUpState_SW/7(a_enum)
  [VPMM_PowerUpState_enum] -> Switch2/1
  Switch2/1 -> Data Type Conversion28/1
  VPMM_InitPowerUpState_enum/1 -> [VPMM_PowerUpState_enum]
  task_time_s/1 -> [task_time_s]
  VPMM_MCUPrechrgProc_flg/1 -> [VPMM_MCUPrechrgProc_flg]
  VPMM_MCUEnableProc_flg/1 -> [VPMM_MCUEnableProc_flg]
  VPMM_DCDCEnableProc_flg/1 -> [VPMM_DCDCEnableProc_flg]
  VPMM_EHPSEnableProc_flg/1 -> [VPMM_EHPSEnableProc_flg]
  VPMM_CACPresReadyProc_flg/1 -> [VPMM_CACPresReadyProc_flg]
  VPMM_InitPowerDownFault_enum/1 -> [VPMM_PowerDownFault_enum]
  VPMM_InitChrgFault_enum/1 -> [VPMM_ChrgFault_enum]
  Data Type Conversion/1 -> cycle time setting/1(trig_cnt)

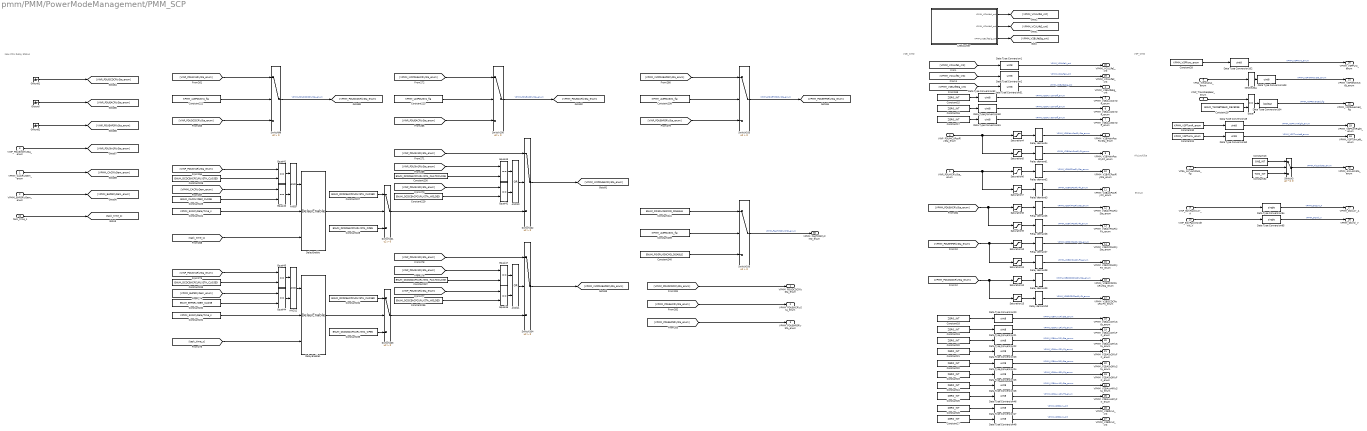
== system pmm/PMM/PowerModeManagement/PMM_SCP ==
  note: EVCU2
  note: AlcLockSta
  note: VSP_CMD
  note: New PCU Relay Status
  note: V2B_CMD
  VPMM_CACRlyDem_enum : Inport
  VPMM_EHPSRlyDem_enum : Inport  Port=2
  VINP_PDU3in1RlySta_enum : Inport  Port=3
  VINP_PDUMCUPosRlySta_enum : Inport  Port=4
  VINP_PDUACRlySta_enum : Inport  Port=5
  VPSA_Keystatus_enum : Inport  Port=6
  VPSA_AlcLockPass_flg : Inport  Port=7
  VINP_TransReqGear_enum : Inport  Port=8
  VINP_B2VPackCurr_A : Inport  Port=9
  VINP_B2VPackInsideVol_V : Inport  Port=10
  task_time_s : Inport  Port=11
  AND10 : Logic  Operator=OR  AllPortsSameDT=off  OutDataTypeStr=boolean
  AND11 : Logic  Operator=OR  AllPortsSameDT=off  OutDataTypeStr=boolean
  AND12 : Logic  AllPortsSameDT=off  OutDataTypeStr=boolean
  AND9 : Logic  AllPortsSameDT=off  OutDataTypeStr=boolean
  Constant13 : Constant  Value=ONE_INT
  Constant{15..27} (13 alike) : Constant  Value=ZERO_INT
  Constant{222..223,238..239} (4 alike) : Constant  Value=KPMM_usePDU3in1_flg
  Constant224 : Constant  Value=KPMM_3in1RlyDelayTime_s
  Constant225 : Constant  Value=ENUM_CACRLYDEM_CLOSE
  Constant{226..227,233..234} (4 alike) : Constant  Value=ENUM_DCDCEACPCURLYSTA_CLOSED
  Constant228 : Constant  Value=ENUM_DCDCEACPCURLYSTA_OPEN
  Constant229 : Constant  Value=ENUM_DCDCEACPCURLYSTA_WELDED
  Constant230 : Constant  Value=ENUM_DCDCEACPCURLYSTA_FAILTOCLOSE
  Constant231 : Constant  Value=KPMM_3in1RlyDelayTime_s
  Constant232 : Constant  Value=ENUM_EHPSRLYDEM_CLOSE
  Constant235 : Constant  Value=ENUM_DCDCEACPCURLYSTA_OPEN
  Constant236 : Constant  Value=ENUM_DCDCEACPCURLYSTA_WELDED
  Constant237 : Constant  Value=ENUM_DCDCEACPCURLYSTA_FAILTOCLOSE
  Constant240 : Constant  Value=ENUM_FOGRLYENCMD_DISABLE
  Constant241 : Constant  Value=ENUM_FOGRLYENCMD_DISABLE
  Constant28 : Constant  Value=KPMM_VSPFunc_enum
  Constant29 : Constant  Value=ENUM_TARGETGEAR_REVERSE
  Constant30 : Constant  Value=KPMM_VSPTurnR_enum
  Constant31 : Constant  Value=KPMM_VSPTurnL_enum
  Constant32 : Constant  Value=TWO_INT
  Data Type Conversion{1..2,20..26,46..52,60..61,102..103} (20 alike) : DataTypeConversion  OutDataTypeStr=uint8
  Data Type Conversion104 : DataTypeConversion  OutDataTypeStr=boolean
  Data Type Conversion94 : DataTypeConversion  OutDataTypeStr=single
  Data Type Conversion95 : DataTypeConversion  OutDataTypeStr=single
  DelayEnable : hcu_lib/Basic_Blocks/DelayEnable
  DelayEnable1 : hcu_lib/Basic_Blocks/DelayEnable
  Equal{,40..47} (9 alike) : RelationalOperator  Operator===  OutDataTypeStr=boolean  RndMeth=Simplest
  Ground : Ground
  Ground1 : Ground
  Ground2 : Ground
  IGNKeySta : LookupNDDirect  NumberOfTableDimensions=1  Table=[0 0 1 ]  TableDataTypeStr=uint8
  LifeCounter : Stateflow chart  TreatAsAtomicUnit=on
  Relay demand{1,3,6,8,10} (5 alike) : LookupNDDirect  NumberOfTableDimensions=1  Table=[0 0 1 2]  TableDataTypeStr=uint8
  Relay demand{2,4..5,7,9} (5 alike) : LookupNDDirect  NumberOfTableDimensions=1  Table=[1 2 0 0]  TableDataTypeStr=uint8
  Saturation{4..13} (10 alike) : Saturate  UpperLimit=3  LowerLimit=0
  Switch{99..106} (8 alike) : Switch  Criteria=u2 > Threshold
  Switch3 : Switch  Criteria=u2 ~= 0
      settings: AttributesFormatString=%<Criteria>
  VPMM_PDUDCDCRlySta_enum : Outport
  VPMM_PDUEACRlySta_enum : Outport  Port=2
  VPMM_PDUEHPSRlySta_enum : Outport  Port=3
  VPMM_V2BLifeSig_cnt : Outport  Port=4
  VPMM_V2BAux1OnOff_enum : Outport  Port=5
  VPMM_V2BAux2OnOff_enum : Outport  Port=6
  VPMM_V2BAux3OnOff_enum : Outport  Port=7
  VPMM_V2BMainPosRlySta_enum : Outport  Port=8
  VPMM_V2BMainPosRlyFit_enum : Outport  Port=9
  VPMM_V2BACPosRlySta_enum : Outport  Port=10
  VPMM_V2BACPosRlyFit_enum : Outport  Port=11
  VPMM_V2BAirPosRlySta_enum : Outport  Port=12
  VPMM_V2BAirPosRlyFit_enum : Outport  Port=13
  VPMM_V2BOilPosRlySta_enum : Outport  Port=14
  VPMM_V2BOilPosRlyFit_enum : Outport  Port=15
  VPMM_V2BDCDCPosRlySta_enum : Outport  Port=16
  VPMM_V2BDCDCPosRlyFit_enum : Outport  Port=17
  VPMM_V2BAux1RlySta_enum : Outport  Port=18
  VPMM_V2BAux1RlyFit_enum : Outport  Port=19
  VPMM_V2BAux2RlySta_enum : Outport  Port=20
  VPMM_V2BAux2RlyFit_enum : Outport  Port=21
  VPMM_V2BAux3RlySta_enum : Outport  Port=22
  VPMM_V2BAux3RlyFit_enum : Outport  Port=23
  VPMM_V2BAux4RlySta_enum : Outport  Port=24
  VPMM_V2BAux4RlyFit_enum : Outport  Port=25
  VPMM_V2BRsv1_cnt : Outport  Port=26
  VPMM_V2BRsv2_cnt : Outport  Port=27
  VPMM_VCULife1_cnt : Outport  Port=28
  VPMM_VCULife2_cnt : Outport  Port=29
  VPMM_VSPFunc_enum : Outport  Port=30
  VPMM_VSPIGNKeySta_enum : Outport  Port=31
  VPMM_VSPReversed_flg : Outport  Port=32
  VPMM_VSPTurnRight_enum : Outport  Port=33
  VPMM_VSPTurnLeft_enum : Outport  Port=34
  VPMM_AlcLockSta_enum : Outport  Port=35
  VPMM_FogTMSRlyCMD_enum : Outport  Port=36
  VPMM_DCCurr_A : Outport  Port=37
  VPMM_DCVol_V : Outport  Port=38
  wires:
  Constant238/1 -> Switch105/2
  Constant231/1 -> DelayEnable1/2
  Constant240/1 -> Switch106/3
  [VPMM_InitPDUEACRlySta_enum] -> Switch100/1
  Switch103/1 -> Switch104/3
  AND10/1 -> Switch102/2
  Ground/1 -> [VINP_PDUEACRlySta_enum]
  Constant229/1 -> Equal42/2
  Switch100/1 -> [VPMM_PDUEACRlySta_enum]  "VPMM_PDUEACRlySta_enum"
  Switch101/1 -> Switch102/3
  Equal43/1 -> AND10/1
  Constant230/1 -> Equal43/2
  VPMM_CACRlyDem_enum/1 -> [VPMM_CACRlyDem_enum]
  Ground2/1 -> [VINP_PDUEHPSRlySta_enum]
  Equal44/1 -> AND12/2
  Switch102/1 -> [VPMM_InitPDUEACRlySta_enum]
  Constant227/1 -> Switch101/1
  Constant232/1 -> Equal44/2
  Switch104/1 -> [VPMM_InitPDUEHPSRlySta_enum]
  Constant235/1 -> Switch103/3
  [VPMM_PDUEACRlySta_enum] -> VPMM_PDUEACRlySta_enum/1
  [VINP_PDU3in1RlySta_enum] -> Equal47/1
  [task_time_s] -> DelayEnable1/3
  Switch99/1 -> [VPMM_PDUDCDCRlySta_enum]  "VPMM_PDUDCDCRlySta_enum"
  DelayEnable/1 -> Switch101/2
  [VPMM_InitPDUEHPSRlySta_enum] -> Switch105/1
  [VINP_PDUEHPSRlySta_enum] -> Switch105/3
  Switch105/1 -> [VPMM_PDUEHPSRlySta_enum]  "VPMM_PDUEHPSRlySta_enum"
  [task_time_s] -> DelayEnable/3
  [VPMM_EHPSRlyDem_enum] -> Equal44/1
  [VPMM_PDUEHPSRlySta_enum] -> VPMM_PDUEHPSRlySta_enum/1
  Switch106/1 -> VPMM_FogTMSRlyCMD_enum/1  "VPMM_FogTMSRlyCMD_enum"
  Constant234/1 -> Switch103/1
  [VINP_PDU3in1RlySta_enum] -> Equal46/1
  Equal41/1 -> AND9/1
  Equal47/1 -> AND11/1
  AND12/1 -> DelayEnable1/1
  Constant223/1 -> Switch100/2
  Equal46/1 -> AND11/2
  Equal45/1 -> AND12/1
  Constant224/1 -> DelayEnable/2
  AND11/1 -> Switch104/2
  [VINP_PDU3in1RlySta_enum] -> Equal42/1
  Constant237/1 -> Equal47/2
  Constant239/1 -> Switch106/2
  VINP_PDU3in1RlySta_enum/1 -> [VINP_PDU3in1RlySta_enum]
  Constant225/1 -> Equal40/2
  [VPMM_CACRlyDem_enum] -> Equal40/1
  [VINP_PDUDCDCRlySta_enum] -> Switch99/3
  [VINP_PDU3in1RlySta_enum] -> Switch99/1
  Equal42/1 -> AND10/2
  Constant222/1 -> Switch99/2
  [VPMM_PDUDCDCRlySta_enum] -> VPMM_PDUDCDCRlySta_enum/1
  Constant226/1 -> Equal41/2
  Constant241/1 -> Switch106/1
  Constant236/1 -> Equal46/2
  AND9/1 -> DelayEnable/1
  Ground1/1 -> [VINP_PDUDCDCRlySta_enum]
  VPMM_EHPSRlyDem_enum/1 -> [VPMM_EHPSRlyDem_enum]
  Constant233/1 -> Equal45/2
  [VINP_PDU3in1RlySta_enum] -> Equal41/1
  [VINP_PDU3in1RlySta_enum] -> Switch102/1
  [VINP_PDU3in1RlySta_enum] -> Equal45/1
  [VINP_PDUEACRlySta_enum] -> Switch100/3
  Equal40/1 -> AND9/2
  [VINP_PDU3in1RlySta_enum] -> Switch104/1
  Constant228/1 -> Switch101/3
  [VINP_PDU3in1RlySta_enum] -> Equal43/1
  DelayEnable1/1 -> Switch103/2
  Saturation8/1 -> Relay demand5/1
  Constant26/1 -> Data Type Conversion47/1
  Saturation10/1 -> Relay demand7/1
  Constant21/1 -> Data Type Conversion23/1
  Relay demand1/1 -> VPMM_V2BMainPosRlyFit_enum/1  "VPMM_V2BMainPosRlyFit_enum"
  Saturation9/1 -> Relay demand6/1
  Constant25/1 -> Data Type Conversion46/1
  Data Type Conversion46/1 -> VPMM_V2BAux4RlyFit_enum/1  "VPMM_V2BAux4RlyFit_enum"
  Constant16/1 -> Data Type Conversion60/1
  Data Type Conversion52/1 -> VPMM_V2BAux1OnOff_enum/1  "VPMM_V2BAux1OnOff_enum"
  Data Type Conversion60/1 -> VPMM_V2BAux2OnOff_enum/1  "VPMM_V2BAux2OnOff_enum"
  Relay demand5/1 -> VPMM_V2BAirPosRlySta_enum/1  "VPMM_V2BAirPosRlySta_enum"
  Data Type Conversion20/1 -> VPMM_V2BAux1RlySta_enum/1  "VPMM_V2BAux1RlySta_enum"
  Data Type Conversion51/1 -> VPMM_V2BLifeSig_cnt/1  "VPMM_V2BLifeSig_cnt"
  Data Type Conversion47/1 -> VPMM_V2BRsv1_cnt/1  "VPMM_V2BRsv1_cnt"
  Saturation5/1 -> Relay demand1/1
  Data Type Conversion25/1 -> VPMM_V2BAux3RlyFit_enum/1  "VPMM_V2BAux3RlyFit_enum"
  Constant20/1 -> Data Type Conversion22/1
  Data Type Conversion61/1 -> VPMM_V2BAux3OnOff_enum/1  "VPMM_V2BAux3OnOff_enum"
  Relay demand8/1 -> VPMM_V2BOilPosRlyFit_enum/1  "VPMM_V2BOilPosRlyFit_enum"
  Constant19/1 -> Data Type Conversion21/1
  Relay demand3/1 -> VPMM_V2BACPosRlyFit_enum/1  "VPMM_V2BACPosRlyFit_enum"
  Relay demand9/1 -> VPMM_V2BDCDCPosRlySta_enum/1  "VPMM_V2BDCDCPosRlySta_enum"
  [VPMM_V2BLifeSig_cnt] -> Data Type Conversion51/1
  Relay demand6/1 -> VPMM_V2BAirPosRlyFit_enum/1  "VPMM_V2BAirPosRlyFit_enum"
  Constant22/1 -> Data Type Conversion24/1
  Data Type Conversion22/1 -> VPMM_V2BAux2RlySta_enum/1  "VPMM_V2BAux2RlySta_enum"
  Data Type Conversion24/1 -> VPMM_V2BAux3RlySta_enum/1  "VPMM_V2BAux3RlySta_enum"
  Constant24/1 -> Data Type Conversion26/1
  Data Type Conversion23/1 -> VPMM_V2BAux2RlyFit_enum/1  "VPMM_V2BAux2RlyFit_enum"
  Constant27/1 -> Data Type Conversion48/1
  Saturation11/1 -> Relay demand8/1
  Saturation7/1 -> Relay demand3/1
  Data Type Conversion26/1 -> VPMM_V2BAux4RlySta_enum/1  "VPMM_V2BAux4RlySta_enum"
  Constant15/1 -> Data Type Conversion52/1
  Relay demand2/1 -> VPMM_V2BACPosRlySta_enum/1  "VPMM_V2BACPosRlySta_enum"
  Relay demand7/1 -> VPMM_V2BOilPosRlySta_enum/1  "VPMM_V2BOilPosRlySta_enum"
  Saturation13/1 -> Relay demand10/1
  Relay demand10/1 -> VPMM_V2BDCDCPosRlyFit_enum/1  "VPMM_V2BDCDCPosRlyFit_enum"
  [VPMM_PDUEACRlySta_enum] -> Saturation9/1, Saturation8/1
  Relay demand4/1 -> VPMM_V2BMainPosRlySta_enum/1  "VPMM_V2BMainPosRlySta_enum"
  Data Type Conversion21/1 -> VPMM_V2BAux1RlyFit_enum/1  "VPMM_V2BAux1RlyFit_enum"
  Constant18/1 -> Data Type Conversion20/1
  Saturation12/1 -> Relay demand9/1
  Constant23/1 -> Data Type Conversion25/1
  Data Type Conversion48/1 -> VPMM_V2BRsv2_cnt/1  "VPMM_V2BRsv2_cnt"
  Saturation4/1 -> Relay demand4/1
  Saturation6/1 -> Relay demand2/1
  Constant17/1 -> Data Type Conversion61/1
  VINP_PDUMCUPosRlySta_enum/1 -> Saturation5/1, Saturation4/1
  VINP_PDUACRlySta_enum/1 -> Saturation7/1, Saturation6/1
  LifeCounter/3(VPMM_V2BLifeSig_cnt) -> [VPMM_V2BLifeSig_cnt]
  [VPMM_PDUEHPSRlySta_enum] -> Saturation11/1, Saturation10/1
  [VPMM_PDUDCDCRlySta_enum] -> Saturation13/1, Saturation12/1
  LifeCounter/1(VPMM_VCULife1_cnt) -> [VPMM_VCULife1_cnt]
  LifeCounter/2(VPMM_VCULife2_cnt) -> [VPMM_VCULife2_cnt]
  Data Type Conversion2/1 -> VPMM_VCULife2_cnt/1  "VPMM_VCULife2_cnt"
  [VPMM_VCULife1_cnt] -> Data Type Conversion1/1
  [VPMM_VCULife2_cnt] -> Data Type Conversion2/1
  Constant28/1 -> Data Type Conversion102/1
  Data Type Conversion102/1 -> VPMM_VSPFunc_enum/1  "VPMM_VSPFunc_enum"
  VPSA_Keystatus_enum/1 -> IGNKeySta/1
  IGNKeySta/1 -> Data Type Conversion103/1
  Data Type Conversion103/1 -> VPMM_VSPIGNKeySta_enum/1  "VPMM_VSPIGNKeySta_enum"
  Data Type Conversion50/1 -> VPMM_VSPTurnLeft_enum/1  "VPMM_VSPTurnLeft_enum"
  Data Type Conversion104/1 -> VPMM_VSPReversed_flg/1  "VPMM_VSPReversed_flg"
  Data Type Conversion49/1 -> VPMM_VSPTurnRight_enum/1  "VPMM_VSPTurnRight_enum"
  Constant30/1 -> Data Type Conversion49/1
  Constant29/1 -> Equal/2
  Equal/1 -> Data Type Conversion104/1
  Constant31/1 -> Data Type Conversion50/1
  Data Type Conversion1/1 -> VPMM_VCULife1_cnt/1  "VPMM_VCULife1_cnt"
  Constant13/1 -> Switch3/1
  Constant32/1 -> Switch3/3
  Switch3/1 -> VPMM_AlcLockSta_enum/1  "VPMM_AlcLockSta_enum"
  VPSA_AlcLockPass_flg/1 -> Switch3/2
  VINP_TransReqGear_enum/1 -> Equal/1
  VINP_B2VPackInsideVol_V/1 -> Data Type Conversion95/1
  Data Type Conversion95/1 -> VPMM_DCVol_V/1  "VPMM_DCVol_V"
  VINP_B2VPackCurr_A/1 -> Data Type Conversion94/1
  Data Type Conversion94/1 -> VPMM_DCCurr_A/1  "VPMM_DCCurr_A"
  task_time_s/1 -> [task_time_s]

== system pmm/PMM/PowerModeManagement/PMM Flag Creator /Alcohole Lock  ==
  VINP_AlcLockSta_flg : Inport
  VDSC_WineDetectorSwitch_flg : Inport  Port=2
  VDMM_DTCAlcLockWireFailure_flg : Inport  Port=3
  AND : Logic  AllPortsSameDT=off  OutDataTypeStr=boolean
  Constant43 : Constant  Value=KPMM_AlcLockSta_flg_ovrdval
  Constant55 : Constant  Value=KPMM_AlcLockSta_flg_ovrdflg
  Constant58 : Constant  Value=TRUE
  Data Type Conversion19 : DataTypeConversion
  NOT : Logic  Operator=NOT  AllPortsSameDT=off  OutDataTypeStr=boolean
  Switch4 : Switch  Criteria=u2 > Threshold
  Switch5 : Switch  Criteria=u2 > Threshold
  VPMM_AlcLockSta_flg : Outport  VectorParamsAs1DForOutWhenUnconnected=off
  wires:
  Switch5/1 -> Switch4/3
  Constant43/1 -> Switch4/1
  Data Type Conversion19/1 -> VPMM_AlcLockSta_flg/1  "VPMM_AlcLockSta_flg"
  [VINP_AlcLockSta_flg] -> Switch5/1
  Switch4/1 -> Data Type Conversion19/1
  Constant58/1 -> Switch5/3
  Constant55/1 -> Switch4/2
  VINP_AlcLockSta_flg/1 -> [VINP_AlcLockSta_flg]
  VDSC_WineDetectorSwitch_flg/1 -> [VDSC_WineDetectorSwitch_flg]
  [VDMM_DTCAlcLockWireFailure_flg] -> NOT/1
  AND/1 -> Switch5/2
  NOT/1 -> AND/2
  [VDSC_WineDetectorSwitch_flg] -> AND/1
  VDMM_DTCAlcLockWireFailure_flg/1 -> [VDMM_DTCAlcLockWireFailure_flg]

== system pmm/PMM/PowerModeManagement/PMM Flag Creator /EHPS Initialization ==
  task_time_s : Inport
  VINP_EHPSMotorSpd_rpm : Inport  Port=2
  Abs : Abs
  Add : Sum  Inputs=+-
  Add1 : Sum
  Constant60 : Constant  Value=KPMM_EHPSEnSpdDiv_rpm
  Constant61 : Constant  Value=KPMM_EHPSSpdDem_rpm
  Constant62 : Constant  Value=ZERO_FLOAT
  Constant63 : Constant  Value=KPMM_EHPSIniHoldTime_s
  Relational Operator1 : RelationalOperator  Operator=<=  OutDataTypeStr=boolean  RndMeth=Simplest
  Relational Operator2 : RelationalOperator  OutDataTypeStr=boolean  RndMeth=Simplest
  Switch6 : Switch  Criteria=u2 > Threshold
  Unit Delay2 : UnitDelay  SampleTime=-1  HasFrameUpgradeWarning=on
  VPMM_EHPSIniReady_flg : Outport
  wires:
  [VINP_EHPSMotorSpd_rpm] -> Add/1
  Abs/1 -> Relational Operator1/1
  Constant61/1 -> Add/2
  Add/1 -> Abs/1
  [task_time_s] -> Add1/2
  Unit Delay2/1 -> Add1/1
  Relational Operator1/1 -> Switch6/2
  Constant63/1 -> Relational Operator2/2
  Constant62/1 -> Switch6/3
  Add1/1 -> Switch6/1
  Switch6/1 -> Relational Operator2/1, Unit Delay2/1
  Constant60/1 -> Relational Operator1/2
  Relational Operator2/1 -> VPMM_EHPSIniReady_flg/1  "VPMM_EHPSIniReady_flg"
  VINP_EHPSMotorSpd_rpm/1 -> [VINP_EHPSMotorSpd_rpm]
  task_time_s/1 -> [task_time_s]
